simulink model "Simulink_Bondoi1"  (R2023a)
settings: Solver=VariableStepAuto  StartTime=0.0  StopTime=1000  RelTol=1e-3
values from neighbouring files (symbols this model uses):
  A1 = D1*D2    (= 171)    [Bondoi_Thongso.m]
  A2 = D2*D1    (= 171)    [Bondoi_Thongso.m]
  aB = 3.14*DB*DB/4    (= 0.2826)    [Bondoi_Thongso.m]
  aC = 3.14*DB*DC/4    (= 0.1884)    [Bondoi_Thongso.m]
  CdB = 0.6    [Bondoi_Thongso.m]
  CdC = 0.6    [Bondoi_Thongso.m]
  g = 981    [Bondoi_Thongso.m]
  h1_init = 0    [Bondoi_Thongso.m]
  h2_init = 0    [Bondoi_Thongso.m]
  kp = 3.3    [Bondoi_Thongso.m]
settings Model: Creator=Admin  LastModifiedBy=Asus
settings SolverCC: AlgebraicLoopSolver=TrustRegion
settings DataIOCC: ReturnWorkspaceOutputs=off
settings DebuggingCC: UnconnectedInputMsg=warning  UnconnectedOutputMsg=warning  UnconnectedLineMsg=warning  ArithmeticOperatorsInVariantConditions=warning
settings ModelReferenceCC: EnableRefExpFcnMdlSchedulingChecks=on
settings SFSimCC: SimUseLocalCustomCode=off  CustomCodeUndefinedFunction=UseInterfaceOnly
settings RTWCC: RTWUseLocalCustomCode=off

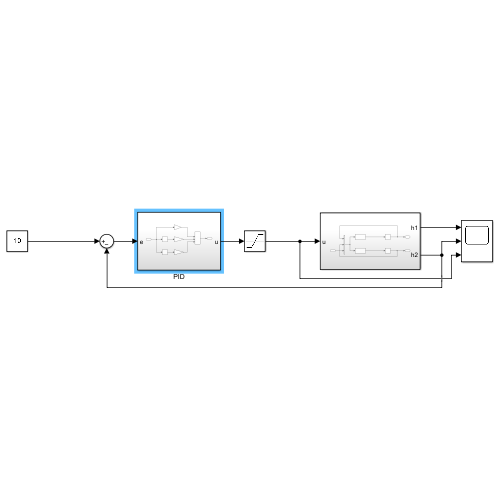
[thumbnail: Simulink's stored preview of the top-level diagram]
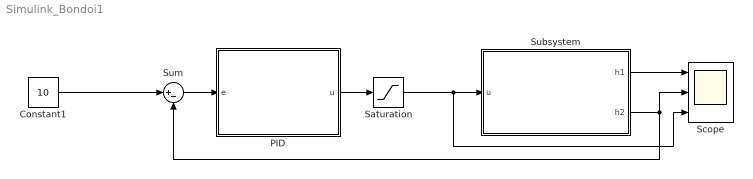
== system Simulink_Bondoi1 ==
  Constant1 : Constant  Value=10
  PID : Subsystem
  Saturation : Saturate  UpperLimit=12  LowerLimit=0
  Scope : Scope  NumInputPorts=3
  Subsystem : Subsystem
  Sum : Sum  Inputs=|+-
  wires:
  Constant1/1 -> Sum/1
  Sum/1 -> PID/1(e)
  PID/1(u) -> Saturation/1
  Saturation/1 -> Scope/3, Subsystem/1(u)
  Subsystem/1(h1) -> Scope/1
  Subsystem/2(h2) -> Sum/2, Scope/2

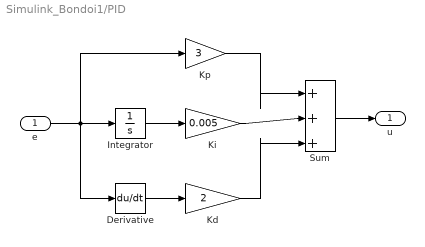
== system Simulink_Bondoi1/PID ==
  e : Inport
  Derivative : Derivative
  Integrator : Integrator
  Kd : Gain  Gain=2
  Ki : Gain  Gain=0.005
  Kp : Gain  Gain=3
  Sum : Sum  Inputs=|+++
  u : Outport  VectorParamsAs1DForOutWhenUnconnected=off
  wires:
  Derivative/1 -> Kd/1
  Sum/1 -> u/1
  Kp/1 -> Sum/1
  Ki/1 -> Sum/2
  Kd/1 -> Sum/3
  Integrator/1 -> Ki/1
  e/1 -> Kp/1, Derivative/1, Integrator/1

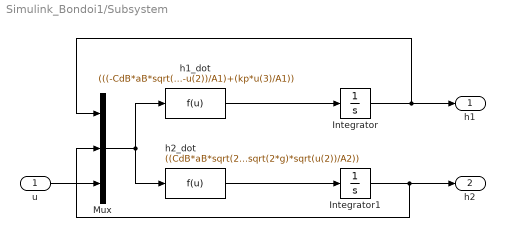
== system Simulink_Bondoi1/Subsystem ==
  u : Inport
  Integrator : Integrator  InitialCondition=h1_init
  Integrator1 : Integrator  InitialCondition=h2_init
  Mux : Mux  Inputs=3
  h1_dot : Fcn  Expr=(((-CdB*aB*sqrt(2*g))*sqrt(u(1)-u(2))/A1)+(kp*u(3)/A1))
  h2_dot : Fcn  Expr=((CdB*aB*sqrt(2*g)*sqrt(u(1)-u(2))/A2)-(CdC*aC*sqrt(2*g)*sqrt(u(2))/A2))
  h1 : Outport  VectorParamsAs1DForOutWhenUnconnected=off
  h2 : Outport  Port=2  VectorParamsAs1DForOutWhenUnconnected=off
  wires:
  Mux/1 -> h2_dot/1, h1_dot/1
  h1_dot/1 -> Integrator/1
  h2_dot/1 -> Integrator1/1
  Integrator/1 -> Mux/1, h1/1
  Integrator1/1 -> Mux/2, h2/1
  u/1 -> Mux/3
